simulink model "pos_pid_simu"  (R2020b)
settings: Solver=VariableStepAuto  StartTime=0.0  StopTime=tfinal  RelTol=1e-3
values from neighbouring files (symbols this model uses):
  Kd = 0    [pos_id_verify.m]    (also in pos_pid_mbd.m = -((p1+p2+p3)*T+1)/K)
  Ki = 0    [pos_id_verify.m]    (also in pos_pid_mbd.m = -p1*p2*p3*T/K)
  Kp = Kp_id    [pos_id_verify.m]    (also in pos_pid_mbd.m = (p1*p2+p2*p3+p3*p1)*T/K)
  r = 60    [pos_id_step.m]
  r_cyc = 8    [pos_id_step.m]
  ts = 1/50    (= 0.02)    [pos_id_step.m]    (also in pos_id_step_fit.m; pos_id_verify.m; pos_pid_mbd.m)
undefined symbols (not defined in the file or in its folder): dend, DiscIntNeverNeededParam, numd
libraries: arduino_io_lib x5, simulink x2
settings Model: Creator=kei55  LastModifiedBy=kei55

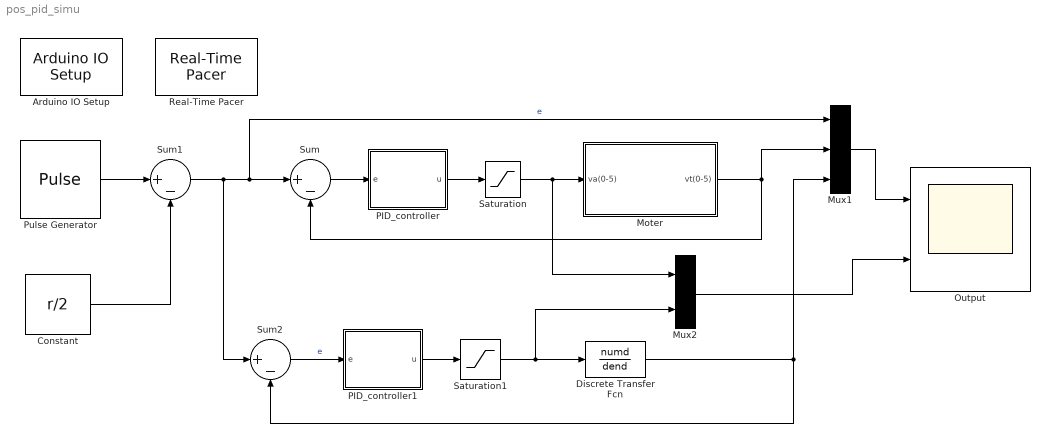
== system pos_pid_simu ==
  Arduino IO Setup : arduino_io_lib/Arduino IO Setup  Priority=3  arduinoVar=Temporary arduino variable: Arduino1  workspaceVarName=a  comPort=COM3
  Constant : Constant  Value=r/2
  Discrete Transfer Fcn : DiscreteTransferFcn  Numerator=numd  Denominator=dend  SampleTime=ts
  Moter : Subsystem
  Mux1 : Mux  Inputs=3
  Mux2 : Mux  Inputs=2
  Output : Scope  NumInputPorts=2
  PID_controller : Subsystem
  PID_controller1 : Subsystem
  Pulse Generator : DiscretePulseGenerator  PulseType=Time based  Amplitude=r  Period=r_cyc  PulseWidth=50  SampleTime=1/50
  Real-Time Pacer : arduino_io_lib/Real-Time Pacer  simTimePerRealTime=1
  Saturation : Saturate  UpperLimit=5.0  LowerLimit=-5.0
  Saturation1 : Saturate  UpperLimit=5.0  LowerLimit=-5.0
  Sum : Sum  Inputs=|+-
  Sum1 : Sum  Inputs=|+-
  Sum2 : Sum  Inputs=|+-
  wires:
  Pulse Generator/1 -> Sum1/1
  Constant/1 -> Sum1/2
  Sum1/1 -> Sum2/1, Sum/1, Mux1/1  "e"
  Moter/1(vt(0-5)) -> Sum/2, Mux1/2
  PID_controller/1(u) -> Saturation/1
  Mux1/1 -> Output/1
  Saturation/1 -> Mux2/1, Moter/1(va(0-5))
  Mux2/1 -> Output/2
  Sum/1 -> PID_controller/1(e)
  Sum2/1 -> PID_controller1/1(e)  "e"
  PID_controller1/1(u) -> Saturation1/1
  Saturation1/1 -> Discrete Transfer Fcn/1, Mux2/2
  Discrete Transfer Fcn/1 -> Sum2/2, Mux1/3

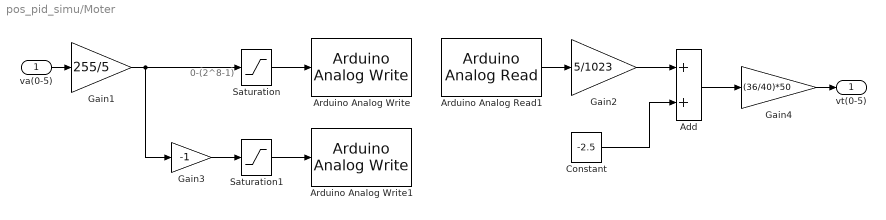
== system pos_pid_simu/Moter ==
  note: 0-(2^8-1)
  va(0-5) : Inport
  Add : Sum
  Arduino Analog Read1 : arduino_io_lib/Arduino Analog Read  arduinoVar=Temporary arduino variable: Arduino1  arduinoPin=0  T=1/50
  Arduino Analog Write : arduino_io_lib/Arduino Analog Write  arduinoVar=Temporary arduino variable: Arduino1  arduinoPin=3  T=1/50
  Arduino Analog Write1 : arduino_io_lib/Arduino Analog Write  arduinoVar=Temporary arduino variable: Arduino1  arduinoPin=5  T=1/50
  Constant : Constant  Value=-2.5
  Gain1 : Gain  Gain=255/5
  Gain2 : Gain  Gain=5/1023
  Gain3 : Gain  Gain=-1
  Gain4 : Gain  Gain=(36/40)*50
  Saturation : Saturate  UpperLimit=255  LowerLimit=0
  Saturation1 : Saturate  UpperLimit=255  LowerLimit=0
  vt(0-5) : Outport
  wires:
  Arduino Analog Read1/1 -> Gain2/1
  va(0-5)/1 -> Gain1/1
  Saturation/1 -> Arduino Analog Write/1
  Saturation1/1 -> Arduino Analog Write1/1
  Gain1/1 -> Gain3/1, Saturation/1
  Gain3/1 -> Saturation1/1
  Gain4/1 -> vt(0-5)/1
  Gain2/1 -> Add/1
  Constant/1 -> Add/2
  Add/1 -> Gain4/1

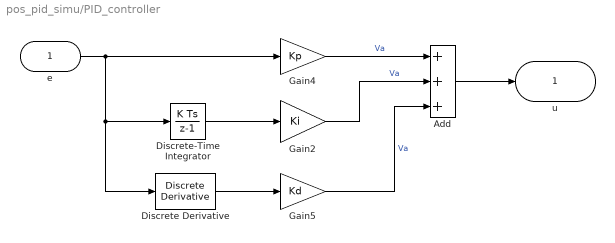
== system pos_pid_simu/PID_controller ==
  e : Inport
  Add : Sum  Inputs=+++
  Discrete Derivative : simulink/Discrete/Discrete Derivative  gainval=1.0  ICPrevScaledInput=0.0  OutMin=[]  OutMax=[]  OutDataType=fixdt(1, 16)  OutScaling=2^-10  DoSatur=off
  Discrete-Time Integrator : DiscreteIntegrator  SampleTime=ts  ICPrevOutput=DiscIntNeverNeededParam  ICPrevScaledInput=DiscIntNeverNeededParam
  Gain2 : Gain  Gain=Ki
  Gain4 : Gain  Gain=Kp
  Gain5 : Gain  Gain=Kd
  u : Outport
  wires:
  Add/1 -> u/1
  Discrete-Time Integrator/1 -> Gain2/1
  e/1 -> Discrete-Time Integrator/1, Discrete Derivative/1, Gain4/1
  Gain4/1 -> Add/1  "Va"
  Gain2/1 -> Add/2  "Va"
  Gain5/1 -> Add/3  "Va"
  Discrete Derivative/1 -> Gain5/1

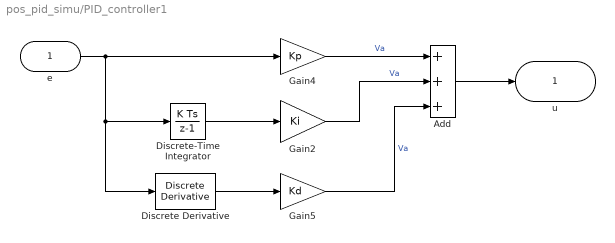
== system pos_pid_simu/PID_controller1 ==
  e : Inport
  Add : Sum  Inputs=+++
  Discrete Derivative : simulink/Discrete/Discrete Derivative  gainval=1.0  ICPrevScaledInput=0.0  OutMin=[]  OutMax=[]  OutDataType=fixdt(1, 16)  OutScaling=2^-10  DoSatur=off
  Discrete-Time Integrator : DiscreteIntegrator  SampleTime=ts  ICPrevOutput=DiscIntNeverNeededParam  ICPrevScaledInput=DiscIntNeverNeededParam
  Gain2 : Gain  Gain=Ki
  Gain4 : Gain  Gain=Kp
  Gain5 : Gain  Gain=Kd
  u : Outport
  wires:
  Discrete Derivative/1 -> Gain5/1
  Gain5/1 -> Add/3  "Va"
  Gain2/1 -> Add/2  "Va"
  Gain4/1 -> Add/1  "Va"
  e/1 -> Gain4/1, Discrete Derivative/1, Discrete-Time Integrator/1
  Discrete-Time Integrator/1 -> Gain2/1
  Add/1 -> u/1
